simulink model "simulink_app"  (R2015a)
settings: Solver=ode2  SolverMode=SingleTasking  StartTime=0.0  StopTime=inf  FixedStep=T_ctrl  RelTol=1e-3
undefined symbols (not defined in the file): A_l_max_x, A_l_max_y, A_z_max, B_hover_4dof, CG_0, epsilon, eta_23, g, h, h_M, Hover_eta_23, Hover_throtle_1, Hover_throtle_23, I_BAC_0, Ix, Iy, Iz, l, l_arm, m, m_0, m_M, Rotation_sign, T_ctrl, throtle_1, throtle_23, v_i0
libraries: XXCopter_Control x52, simulink x11, XXCopter x1
(part 2 of 4)

== system simulink_app/Control and guidance/Otter Overactuated P Controller ==
  Position ref (m) : Inport
  Vel_yaw_ref(m) : Inport  Port=2
  All meas : Inport  Port=3
  activation_bus : Inport  Port=4
  init_cond : Inport  Port=5
  AWU : Product  Multiplication=Matrix(*)
  Add : Sum
  Add1 : Sum  Inputs=+-
  Add2 : Sum  Inputs=+-
  Bus Selector1 : BusSelector  OutputSignals=Params.T_Fe_Fyaw,Params.V_yaw,Params.DCM
  Bus Selector2 : BusSelector  OutputSignals=pos_xy_act,vel_yaw_xy_act,alt_act,vel_yaw_z_act
  Demux1 : Demux  Outputs=3
  Demux2 : Demux  Outputs=3
  Demux3 : Demux  Outputs=[2,1]
  Logical Operator : Logic  IconShape=distinctive  AllPortsSameDT=off  OutDataTypeStr=boolean
  Logical Operator1 : Logic  Operator=NOT  IconShape=distinctive  AllPortsSameDT=off  OutDataTypeStr=boolean
  Logical Operator2 : Logic  Operator=NOT  IconShape=distinctive  AllPortsSameDT=off  OutDataTypeStr=boolean
  Logical Operator3 : Logic  IconShape=distinctive  AllPortsSameDT=off  OutDataTypeStr=boolean
  Matrix Multiply1 : Product  Multiplication=Matrix(*)
  Matrix Multiply2 : Product  Multiplication=Matrix(*)
  Matrix Multiply3 : Product  Multiplication=Matrix(*)
  Memory : Memory  X0=[0;0;0]  InheritSampleTime=on
  Mux : Mux  Inputs=[2,1]
  Permute Dimensions : PermuteDimensions
  Permute Dimensions1 : PermuteDimensions
  Permute Dimensions2 : PermuteDimensions
  Position Controller : Subsystem
  Saturation : Saturate  UpperLimit=[A_l_max_x,A_l_max_y,g]  LowerLimit=-[A_l_max_x,A_l_max_y,A_z_max-g]
  Saturation1 : Saturate  UpperLimit=[10,10,v_i0]'  LowerLimit=-[10,10,2*v_i0]'
  Selector : Selector  InputPortWidth=3  Indices=[1,2]
  Selector1 : Selector  InputPortWidth=3  Indices=3
  Switch : Switch  Criteria=u2 ~= 0
  Switch1 : Switch  Criteria=u2 ~= 0
  T : Gain  Gain=T_ctrl
  Velocity Controller : Subsystem
  activation_bus1 : InportShadow  Port=4
  init_cond1 : InportShadow  Port=5
  Accels des : Outport
  wires:
  Demux2/3 -> Velocity Controller/3(Vyaw_z_ref)
  Demux2/1 -> Velocity Controller/1(Vyaw_x_ref)
  Demux2/2 -> Velocity Controller/2(Vyaw_y_ref)
  All meas/1 -> Position Controller/6(All_meas), Bus Selector1/1
  Position ref (m)/1 -> Demux1/1
  Demux1/3 -> Position Controller/4(X_e_z_ref)
  Demux1/2 -> Position Controller/3(X_e_y_ref)
  Demux1/1 -> Position Controller/2(X_e_x_ref)
  Bus Selector1/3 -> Permute Dimensions/1  "<DCM>"
  Matrix Multiply1/1 -> Accels des/1
  Permute Dimensions/1 -> Matrix Multiply1/1
  Position Controller/1(Ve des (m/s)) -> Matrix Multiply2/2
  Saturation1/1 -> Add1/1, Demux2/1
  Saturation/1 -> Add2/1, Matrix Multiply3/2
  Bus Selector1/1 -> Permute Dimensions2/1, Matrix Multiply2/1, Permute Dimensions1/1  "<T_Fe_Fyaw>"
  Mux/1 -> Add1/2, Saturation1/1
  Matrix Multiply3/1 -> Matrix Multiply1/2  "in F_e"
  Permute Dimensions1/1 -> Matrix Multiply3/1
  Velocity Controller/1(Acc_yaw des (m/s)) -> Add2/2, Saturation/1
  Permute Dimensions2/1 -> AWU/1
  Add/1 -> AWU/2
  Add2/1 -> T/1
  Add1/1 -> Add/2
  AWU/1 -> Memory/1
  T/1 -> Add/1
  activation_bus/1 -> Bus Selector2/1, Position Controller/5(activation_bus)
  activation_bus1/1 -> Velocity Controller/5(activation_bus)
  init_cond/1 -> Position Controller/7(init_cond)
  Bus Selector1/2 -> Velocity Controller/4(V_yaw_meas)  "<V_yaw>"
  Matrix Multiply2/1 -> Demux3/1
  Switch/1 -> Mux/1
  Demux3/1 -> Switch/3
  Vel_yaw_ref(m)/1 -> Selector/1, Selector1/1
  Selector/1 -> Switch/1
  Switch1/1 -> Mux/2
  Demux3/2 -> Switch1/3
  Selector1/1 -> Switch1/1
  init_cond1/1 -> Velocity Controller/6(Init_cond)
  Bus Selector2/1 -> Logical Operator1/1  "<pos_xy_act>"
  Bus Selector2/3 -> Logical Operator2/1  "<alt_act>"
  Logical Operator1/1 -> Logical Operator/1
  Bus Selector2/2 -> Logical Operator/2  "<vel_yaw_xy_act>"
  Logical Operator2/1 -> Logical Operator3/1
  Bus Selector2/4 -> Logical Operator3/2  "<vel_yaw_z_act>"
  Logical Operator/1 -> Switch/2
  Logical Operator3/1 -> Switch1/2
  Memory/1 -> Position Controller/1(AWU)

== system simulink_app/Control and guidance/keep -90//90 ==
  in (rad) : Inport
  Constant : Constant  Value=180
  Constant2 : Constant  Value=360
  Gain : Gain  Gain=360
  Math Function2 : Math  Operator=rem  SaturateOnIntegerOverflow=on
  Product : Product  Inputs=*/  RndMeth=Zero
  Rounding Function : Rounding  Operator=fix
  Sum2 : Sum  Inputs=|-+
  deg2rad1 : Gain  Gain=pi/180  SaturateOnIntegerOverflow=on  OutDataTypeStr=Inherit: Same as input  ParamDataTypeStr=Inherit: Same as input
  rad2deg : Gain  Gain=180/pi  SaturateOnIntegerOverflow=on  OutDataTypeStr=Inherit: Same as input  ParamDataTypeStr=Inherit: Same as input
  out (rad) : Outport
  wires:
  deg2rad1/1 -> out (rad)/1
  Sum2/1 -> deg2rad1/1
  Math Function2/1 -> Sum2/2, Product/1
  Constant2/1 -> Math Function2/2
  rad2deg/1 -> Math Function2/1
  Gain/1 -> Sum2/1
  Rounding Function/1 -> Gain/1
  Product/1 -> Rounding Function/1
  Constant/1 -> Product/2
  in (rad)/1 -> rad2deg/1

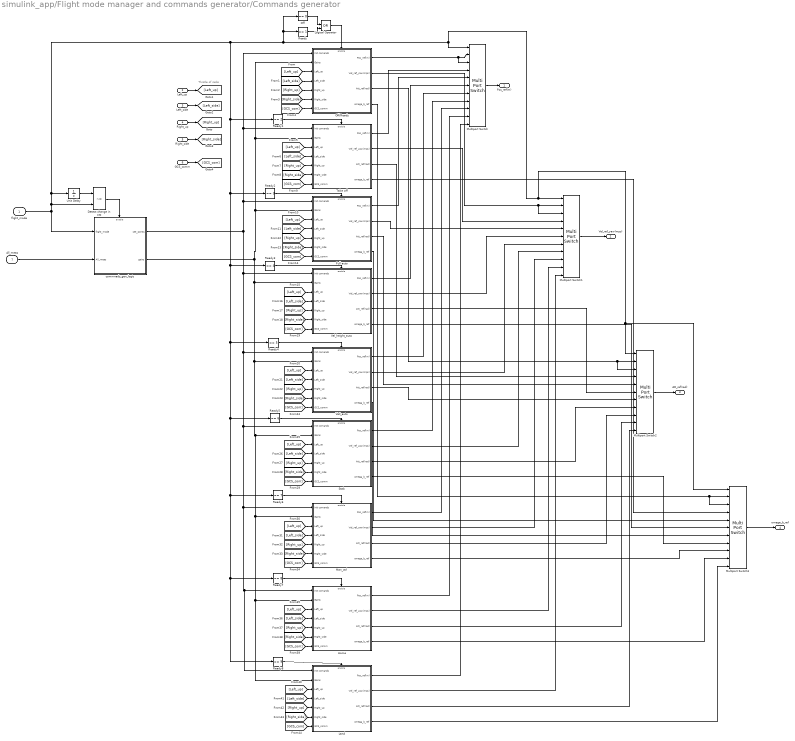
== system simulink_app/Flight mode manager and commands generator/Commands generator ==
  note: Throtle of radio
  flight_mode : Inport
  Left_up : Inport  Port=2
  Left_side : Inport  Port=3
  Right_up : Inport  Port=4
  Right_side : Inport  Port=5
  GCS_comm : Inport  Port=6
  All_meas : Inport  Port=7
  Detect change in FM : RelationalOperator  Operator=~=  OutDataTypeStr=boolean
  Full auto : Subsystem  TreatAsAtomicUnit=on
  Home : Subsystem  TreatAsAtomicUnit=on
  "Land " : Subsystem  TreatAsAtomicUnit=on
  Logical Operator : Logic  Operator=OR  IconShape=distinctive  AllPortsSameDT=off  OutDataTypeStr=boolean
  Man_ctrl : Subsystem  TreatAsAtomicUnit=on
  Multiport Switch{,1..3} (4 alike) : MultiPortSwitch  DataPortOrder=Zero-based contiguous  Inputs=10
  Off : simulink/Logic and Bit Operations/Compare To Constant  relop===  const=0  OutDataTypeStr=boolean
  Off/Ready : Subsystem  TreatAsAtomicUnit=on
  Ready : simulink/Logic and Bit Operations/Compare To Constant  relop===  const=1  OutDataTypeStr=boolean
  Ready1 : simulink/Logic and Bit Operations/Compare To Constant  relop===  const=2  OutDataTypeStr=boolean
  Ready2 : simulink/Logic and Bit Operations/Compare To Constant  relop===  const=3  OutDataTypeStr=boolean
  Ready3 : simulink/Logic and Bit Operations/Compare To Constant  relop===  const=4  OutDataTypeStr=boolean
  Ready4 : simulink/Logic and Bit Operations/Compare To Constant  relop===  const=5  OutDataTypeStr=boolean
  Ready5 : simulink/Logic and Bit Operations/Compare To Constant  relop===  const=6  OutDataTypeStr=boolean
  Ready6 : simulink/Logic and Bit Operations/Compare To Constant  relop===  const=7  OutDataTypeStr=boolean
  Ready7 : simulink/Logic and Bit Operations/Compare To Constant  relop===  const=8  OutDataTypeStr=boolean
  Ready8 : simulink/Logic and Bit Operations/Compare To Constant  relop===  const=9  OutDataTypeStr=boolean
  Stab : Subsystem  TreatAsAtomicUnit=on
  Take off : Subsystem  TreatAsAtomicUnit=on
  Unit Delay : UnitDelay  SampleTime=-1
  Vel_height_auto : Subsystem  TreatAsAtomicUnit=on
  Vell_auto : Subsystem  TreatAsAtomicUnit=on
  commnads_gen_logic : Subsystem
  Pos_ref(m) : Outport
  Vel_ref_yaw(mps) : Outport  Port=2
  Att_ref(rad) : Outport  Port=3
  omega_b_ref : Outport  Port=4
  wires:
  flight_mode/1 -> Detect change in FM/2, Unit Delay/1, Ready8/1, Ready7/1, Ready6/1, Ready5/1, Ready4/1, Ready3/1, Ready2/1, Ready1/1, Ready/1, Off/1, Multiport Switch2/1, Multiport Switch3/1, Multiport Switch1/1, Multiport Switch/1, commnads_gen_logic/1(flight_mode)
  Multiport Switch/1 -> Pos_ref(m)/1
  Multiport Switch1/1 -> Vel_ref_yaw(mps)/1
  Multiport Switch2/1 -> Att_ref(rad)/1
  Multiport Switch3/1 -> omega_b_ref/1
  Right_up/1 -> [Right_up]
  Left_up/1 -> [Left_up]
  Right_side/1 -> [Right_side]
  Left_side/1 -> [Left_side]
  GCS_comm/1 -> [GCS_com]
  [Left_up] -> Off/Ready/3(Left_up)
  [Left_side] -> Off/Ready/4(Left_side)
  [Right_up] -> Off/Ready/5(Right_up)
  [Right_side] -> Off/Ready/6(Right_side)
  [GCS_com] -> Off/Ready/7(GCS_comm)
  [Left_up] -> Take off/3(Left_up)
  [Left_side] -> Take off/4(Left_side)
  [Right_up] -> Take off/5(Right_up)
  [Right_side] -> Take off/6(Right_side)
  [GCS_com] -> Take off/7(GCS_comm)
  [Left_up] -> Full auto/3(Left_up)
  [Left_side] -> Full auto/4(Left_side)
  [Right_up] -> Full auto/5(Right_up)
  [Right_side] -> Full auto/6(Right_side)
  [GCS_com] -> Full auto/7(GCS_comm)
  [Left_up] -> Vel_height_auto/3(Left_up)
  [Left_side] -> Vel_height_auto/4(Left_side)
  [Right_up] -> Vel_height_auto/5(Right_up)
  [Right_side] -> Vel_height_auto/6(Right_side)
  [GCS_com] -> Vel_height_auto/7(GCS_comm)
  [Left_up] -> Vell_auto/3(Left_up)
  [Left_side] -> Vell_auto/4(Left_side)
  [Right_up] -> Vell_auto/5(Right_up)
  [Right_side] -> Vell_auto/6(Right_side)
  [GCS_com] -> Vell_auto/7(GCS_comm)
  [Left_up] -> Stab/3(Left_up)
  [Left_side] -> Stab/4(Left_side)
  [Right_up] -> Stab/5(Right_up)
  [Right_side] -> Stab/6(Right_side)
  [GCS_com] -> Stab/7(GCS_comm)
  [Left_up] -> Man_ctrl/3(Left_up)
  [Left_side] -> Man_ctrl/4(Left_side)
  [Right_up] -> Man_ctrl/5(Right_up)
  [Right_side] -> Man_ctrl/6(Right_side)
  [GCS_com] -> Man_ctrl/7(GCS_comm)
  [Left_up] -> Home/3(Left_up)
  [Left_side] -> Home/4(Left_side)
  [Right_up] -> Home/5(Right_up)
  [Right_side] -> Home/6(Right_side)
  [GCS_com] -> Home/7(GCS_comm)
  [Left_up] -> "Land "/3(Left_up)
  [Left_side] -> "Land "/4(Left_side)
  [Right_up] -> "Land "/5(Right_up)
  [Right_side] -> "Land "/6(Right_side)
  [GCS_com] -> "Land "/7(GCS_comm)
  Off/1 -> Logical Operator/1
  Ready/1 -> Logical Operator/2
  Logical Operator/1 -> Off/Ready/Enable
  Ready1/1 -> Take off/Enable
  Ready2/1 -> Full auto/Enable
  Ready3/1 -> Vel_height_auto/Enable
  Ready4/1 -> Vell_auto/Enable
  Ready5/1 -> Stab/Enable
  Ready6/1 -> Man_ctrl/Enable
  Ready7/1 -> Home/Enable
  Ready8/1 -> "Land "/Enable
  Off/Ready/1(Pos_ref(m)) -> Multiport Switch/3, Multiport Switch/2
  Take off/1(Pos_ref(m)) -> Multiport Switch/4
  Full auto/1(Pos_ref(m)) -> Multiport Switch/5
  Vel_height_auto/1(Pos_ref(m)) -> Multiport Switch/6
  Vell_auto/1(Pos_ref(m)) -> Multiport Switch/7
  Stab/1(Pos_ref(m)) -> Multiport Switch/8
  Man_ctrl/1(Pos_ref(m)) -> Multiport Switch/9
  Home/1(Pos_ref(m)) -> Multiport Switch/10
  "Land "/1(Pos_ref(m)) -> Multiport Switch/11
  Off/Ready/2(Vel_ref_yaw(mps)) -> Multiport Switch1/3, Multiport Switch1/2
  Take off/2(Vel_ref_yaw(mps)) -> Multiport Switch1/4
  Full auto/2(Vel_ref_yaw(mps)) -> Multiport Switch1/5
  Vel_height_auto/2(Vel_ref_yaw(mps)) -> Multiport Switch1/6
  Vell_auto/2(Vel_ref_yaw(mps)) -> Multiport Switch1/7
  Stab/2(Vel_ref_yaw(mps)) -> Multiport Switch1/8
  Man_ctrl/2(Vel_ref_yaw(mps)) -> Multiport Switch1/9
  Home/2(Vel_ref_yaw(mps)) -> Multiport Switch1/10
  "Land "/2(Vel_ref_yaw(mps)) -> Multiport Switch1/11
  Off/Ready/3(Att_ref(rad)) -> Multiport Switch2/3, Multiport Switch2/2
  Take off/3(Att_ref(rad)) -> Multiport Switch2/4
  Full auto/3(Att_ref(rad)) -> Multiport Switch2/5
  Vel_height_auto/3(Att_ref(rad)) -> Multiport Switch2/6
  Vell_auto/3(Att_ref(rad)) -> Multiport Switch2/7
  Stab/3(Att_ref(rad)) -> Multiport Switch2/8
  Man_ctrl/3(Att_ref(rad)) -> Multiport Switch2/9
  Home/3(Att_ref(rad)) -> Multiport Switch2/10
  "Land "/3(Att_ref(rad)) -> Multiport Switch2/11
  Off/Ready/4(omega_b_ref) -> Multiport Switch3/3, Multiport Switch3/2
  Take off/4(omega_b_ref) -> Multiport Switch3/4
  Full auto/4(omega_b_ref) -> Multiport Switch3/5
  Vel_height_auto/4(omega_b_ref) -> Multiport Switch3/6
  Vell_auto/4(omega_b_ref) -> Multiport Switch3/7
  Stab/4(omega_b_ref) -> Multiport Switch3/8
  Man_ctrl/4(omega_b_ref) -> Multiport Switch3/9
  Home/4(omega_b_ref) -> Multiport Switch3/10
  "Land "/4(omega_b_ref) -> Multiport Switch3/11
  commnads_gen_logic/2(gains) -> Full auto/2(Gains), Take off/2(Gains), Off/Ready/2(Gains), Stab/2(Gains), "Land "/2(Gains), Home/2(Gains), Man_ctrl/2(Gains), Vell_auto/2(Gains), Vel_height_auto/2(Gains)
  commnads_gen_logic/1(set_points) -> Take off/1(Init comands), Off/Ready/1(Init comands), Full auto/1(Init comands), Stab/1(Init comands), "Land "/1(Init comands), Home/1(Init comands), Man_ctrl/1(Init comands), Vell_auto/1(Init comands), Vel_height_auto/1(Init comands)
  All_meas/1 -> commnads_gen_logic/2(All_meas)
  Unit Delay/1 -> Detect change in FM/1
  Detect change in FM/1 -> commnads_gen_logic/Enable

== system simulink_app/Flight mode manager and commands generator/Flight manager ==
  note: This guy should be able to overwrite any flghlit_mode at any moment
  flight_mode_request : Inport
  All_meas : Inport  Port=2
  Safety_stab_switch : Inport  Port=3
  Bus Selector : BusSelector  OutputSignals=Params.gps_pdop,Params.gps_sat,Meas.Pos_meas_m,Params.V_yaw,Meas.Eulr_meas_rad,Meas.Volt
  Bus Selector1 : BusSelector  OutputSignals=Params.gps_pdop,Params.gps_vdop,Params.gps_sat,Meas.Pos_meas_m,Meas.Volt,Params.a_meas
  Memory : Memory
  Parameters_based_decision_making : MATLAB Function  TreatAsAtomicUnit=on
  Selector : Selector  InputPortWidth=3  Indices=3
  Unary Minus : UnaryMinus
  flight_mode_manager : MATLAB Function  TreatAsAtomicUnit=on
  flight_mode : Outport
  not_allowed_transition : Outport  Port=2
  wires:
  flight_mode_request/1 -> flight_mode_manager/1(flight_mode_reqest)
  All_meas/1 -> Bus Selector1/1, Bus Selector/1
  flight_mode_manager/1(flight_mode_out) -> Parameters_based_decision_making/1(flight_mode)
  Parameters_based_decision_making/1(flight_mode_out) -> flight_mode/1, Memory/1
  Memory/1 -> flight_mode_manager/9(flight_mode)
  Safety_stab_switch/1 -> flight_mode_manager/2(Safety_stab_switch)
  Bus Selector/1 -> flight_mode_manager/3(p_dop)  "<gps_pdop>"
  Bus Selector/5 -> flight_mode_manager/7(Euler)  "<Eulr_meas_rad>"
  Bus Selector/4 -> flight_mode_manager/6(Vyaw)  "<V_yaw>"
  Bus Selector/3 -> flight_mode_manager/5(Xe)  "<Pos_meas_m>"
  Bus Selector/2 -> flight_mode_manager/4(num_sats)  "<gps_sat>"
  Bus Selector1/1 -> Parameters_based_decision_making/2(pdop)  "<gps_pdop>"
  Bus Selector1/2 -> Parameters_based_decision_making/3(vdop)  "<gps_vdop>"
  Bus Selector1/3 -> Parameters_based_decision_making/4(num_sats)  "<gps_sat>"
  Bus Selector1/5 -> Parameters_based_decision_making/6(Volt)  "<Volt>"
  Bus Selector1/6 -> Parameters_based_decision_making/7(Accs)  "<a_meas>"
  Selector/1 -> Unary Minus/1
  Bus Selector1/4 -> Selector/1  "<Pos_meas_m>"
  Unary Minus/1 -> Parameters_based_decision_making/5(Alt)
  Bus Selector/6 -> flight_mode_manager/8(Volt)  "<Volt>"
  flight_mode_manager/2(NOT_allowed_sign) -> not_allowed_transition/1

== system simulink_app/Px4_to_simulink input interface/DCM1 ==
  Euler : Inport  PortDimensions=3
  Fcn11 : Fcn  Expr=u(5)*u(4)
  Fcn12 : Fcn  Expr=u(5)*u(1)
  Fcn13 : Fcn  Expr=-u(2)
  Fcn21 : Fcn  Expr=u(3)*u(2)*u(4) - u(6)*u(1)
  Fcn22 : Fcn  Expr=u(3)*u(2)*u(1) + u(6)*u(4)
  Fcn23 : Fcn  Expr=u(3)*u(5)
  Fcn31 : Fcn  Expr=u(6)*u(2)*u(4) + u(3)*u(1)
  Fcn32 : Fcn  Expr=u(6)*u(2)*u(1) - u(3)*u(4)
  Fcn33 : Fcn  Expr=u(6)*u(5)
  Mux : Mux  Inputs=2
  Mux1 : Mux  Inputs=9
  Reshape : Reshape  OutputDimensionality=Customize  OutputDimensions=[3,3]
  sincos : Trigonometry  Operator=sincos
  DCM : Outport  PortDimensions=[3,3]
  wires:
  Fcn33/1 -> Mux1/9
  Fcn32/1 -> Mux1/8
  Fcn23/1 -> Mux1/6
  Fcn22/1 -> Mux1/5
  Fcn31/1 -> Mux1/7
  Fcn21/1 -> Mux1/4
  Fcn13/1 -> Mux1/3
  Fcn12/1 -> Mux1/2
  Fcn11/1 -> Mux1/1
  Mux/1 -> Fcn22/1, Fcn23/1, Fcn31/1, Fcn33/1, Fcn32/1, Fcn21/1, Fcn13/1, Fcn12/1, Fcn11/1
  sincos/2 -> Mux/2
  sincos/1 -> Mux/1
  Reshape/1 -> DCM/1
  Euler/1 -> sincos/1
  Mux1/1 -> Reshape/1

== system simulink_app/Control and guidance/Control allocator/Hover deflections1 ==
  Contro Inputs1 : Constant  Value=Hover_throtle_1
  Contro Inputs2 : Constant  Value=Hover_throtle_23
  Contro Inputs3 : Constant  Value=Hover_eta_23
  Gain : Gain  Gain=-1
  Ground : Ground
  Mux : Mux  Inputs=9
  Trim deflectins : Outport
  wires:
  Contro Inputs1/1 -> Mux/1
  Contro Inputs2/1 -> Mux/7, Mux/4
  Ground/1 -> Mux/2, Mux/6, Mux/9, Mux/3
  Contro Inputs3/1 -> Gain/1, Mux/5
  Gain/1 -> Mux/8
  Mux/1 -> Trim deflectins/1

== system simulink_app/Control and guidance/Control allocator/Hover deflections2 ==
  Contro Inputs1 : Constant  Value=Hover_throtle_1
  Contro Inputs2 : Constant  Value=Hover_throtle_23
  Contro Inputs3 : Constant  Value=Hover_eta_23
  Gain : Gain  Gain=-1
  Ground : Ground
  Mux : Mux  Inputs=9
  Trim deflectins : Outport
  wires:
  Contro Inputs1/1 -> Mux/1
  Contro Inputs2/1 -> Mux/7, Mux/4
  Ground/1 -> Mux/2, Mux/6, Mux/9, Mux/3
  Contro Inputs3/1 -> Gain/1, Mux/5
  Gain/1 -> Mux/8
  Mux/1 -> Trim deflectins/1

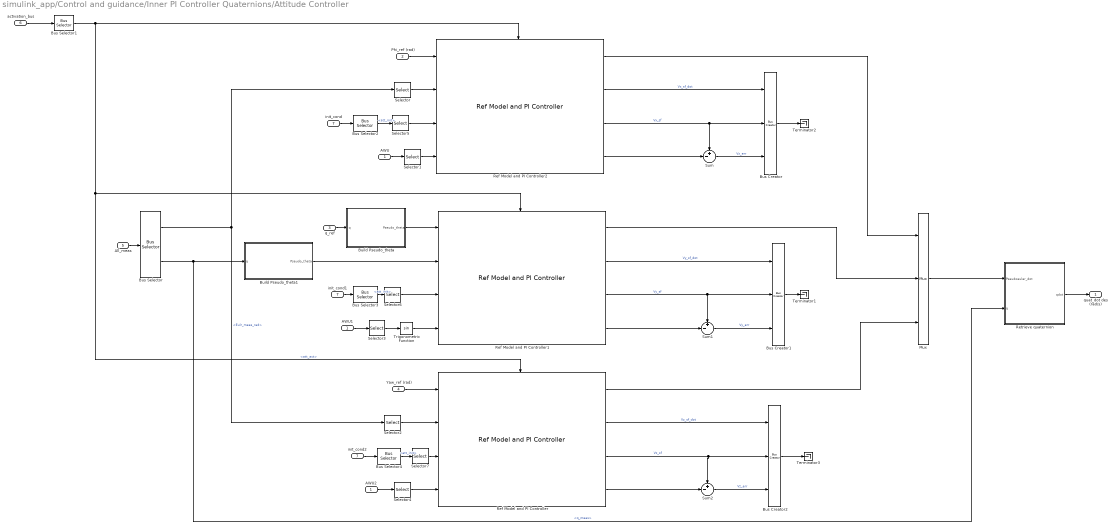
== system simulink_app/Control and guidance/Inner PI Controller Quaternions/Attitude Controller ==
  AWU : Inport
  Phi_ref (rad) : Inport  Port=2
  q_ref : Inport  Port=3
  Yaw_ref (rad) : Inport  Port=4
  All_meas : Inport  Port=5
  activation_bus : Inport  Port=6
  init_cond : Inport  Port=7
  AWU1 : InportShadow
  AWU2 : InportShadow
  Build Pseudo_theta : MATLAB Function  TreatAsAtomicUnit=on
  Build Pseudo_theta1 : MATLAB Function  TreatAsAtomicUnit=on
  Bus Creator : BusCreator  Inputs=3
  Bus Creator1 : BusCreator  Inputs=3
  Bus Creator2 : BusCreator  Inputs=3
  Bus Selector : BusSelector  OutputSignals=Meas.Eulr_meas_rad,Meas.q_meas
  Bus Selector1 : BusSelector  OutputSignals=att_act
  Bus Selector2 : BusSelector  OutputSignals=att_init
  Bus Selector3 : BusSelector  OutputSignals=att_init
  Bus Selector4 : BusSelector  OutputSignals=att_init
  Mux : Mux  Inputs=3
  Ref Model and PI Controller : XXCopter_Control/Ref Model and PI Controller  delta=0  tau=2  RisingSlewLimit=deg2rad(8)  FallingSlewLimit=-deg2rad(8)  K_f=0  K_a=1  Con_way=pro  omega_n=4  xi=0.5  Z1=-30  K_b=2  f_i=0.15  f_c=1
  Ref Model and PI Controller1 : XXCopter_Control/Ref Model and PI Controller  delta=0  tau=1.5  RisingSlewLimit=deg2rad(8)  FallingSlewLimit=-deg2rad(8)  K_f=0  K_a=1  Con_way=pro  omega_n=4  xi=0.5  Z1=-30  K_b=1.2  f_i=0.1  f_c=1
  Ref Model and PI Controller2 : XXCopter_Control/Ref Model and PI Controller  delta=0  tau=1.5  RisingSlewLimit=deg2rad(8)  FallingSlewLimit=-deg2rad(8)  K_f=0  K_a=1  Con_way=pro  omega_n=4  xi=0.5  Z1=-30  K_b=1.5  f_i=0.1  f_c=1
  Retrieve quaternion : MATLAB Function  TreatAsAtomicUnit=on
  Selector : Selector  InputPortWidth=3
  Selector1 : Selector  InputPortWidth=3
  Selector2 : Selector  InputPortWidth=3  Indices=3
  Selector3 : Selector  InputPortWidth=3  Indices=2
  Selector4 : Selector  InputPortWidth=3  Indices=3
  Selector5 : Selector  InputPortWidth=3
  Selector6 : Selector  InputPortWidth=3  Indices=2
  Selector7 : Selector  InputPortWidth=3  Indices=3
  Sum : Sum  Inputs=+-|
  Sum1 : Sum  Inputs=+-|
  Sum2 : Sum  Inputs=+-|
  Terminator1 : Terminator
  Terminator2 : Terminator
  Terminator3 : Terminator
  Trigonometric Function : Trigonometry
  init_cond1 : InportShadow  Port=7
  init_cond2 : InportShadow  Port=7
  quat_dot des (rad/s) : Outport
  wires:
  Ref Model and PI Controller/4 -> Sum2/2
  Sum2/1 -> Bus Creator2/3  "Vz_err"
  Ref Model and PI Controller/3 -> Bus Creator2/2, Sum2/1  "Vz_sf"
  Ref Model and PI Controller/2 -> Bus Creator2/1  "Vz_sf_dot"
  Ref Model and PI Controller1/4 -> Sum1/2
  Sum1/1 -> Bus Creator1/3  "Vy_err"
  Ref Model and PI Controller1/3 -> Bus Creator1/2, Sum1/1  "Vy_sf"
  Ref Model and PI Controller1/2 -> Bus Creator1/1  "Vy_sf_dot"
  Ref Model and PI Controller2/4 -> Sum/2
  Bus Creator2/1 -> Terminator3/1
  Bus Creator1/1 -> Terminator1/1
  Bus Creator/1 -> Terminator2/1
  Sum/1 -> Bus Creator/3  "Vx_err"
  Ref Model and PI Controller2/3 -> Bus Creator/2, Sum/1  "Vx_sf"
  Ref Model and PI Controller2/2 -> Bus Creator/1  "Vx_sf_dot"
  Yaw_ref (rad)/1 -> Ref Model and PI Controller/1
  Selector/1 -> Ref Model and PI Controller2/2
  Bus Selector/2 -> Retrieve quaternion/2(q), Build Pseudo_theta1/1(q)  "<q_meas>"
  All_meas/1 -> Bus Selector/1
  q_ref/1 -> Build Pseudo_theta/1(q)
  Phi_ref (rad)/1 -> Ref Model and PI Controller2/1
  Retrieve quaternion/1(qdot) -> quat_dot des (rad/s)/1
  Ref Model and PI Controller2/1 -> Mux/1
  Ref Model and PI Controller/1 -> Mux/3
  Ref Model and PI Controller1/1 -> Mux/2
  Mux/1 -> Retrieve quaternion/1(Pseudoeuler_dot)
  Selector2/1 -> Ref Model and PI Controller/2
  Bus Selector/1 -> Selector2/1, Selector/1  "<Eulr_meas_rad>"
  Build Pseudo_theta1/1(Pseudo_theta) -> Ref Model and PI Controller1/2
  Build Pseudo_theta/1(Pseudo_theta) -> Ref Model and PI Controller1/1
  AWU/1 -> Selector1/1
  AWU1/1 -> Selector3/1
  AWU2/1 -> Selector4/1
  Selector3/1 -> Trigonometric Function/1
  Selector1/1 -> Ref Model and PI Controller2/4
  Trigonometric Function/1 -> Ref Model and PI Controller1/4
  Selector4/1 -> Ref Model and PI Controller/4
  activation_bus/1 -> Bus Selector1/1
  Bus Selector1/1 -> Ref Model and PI Controller/Enable, Ref Model and PI Controller1/Enable, Ref Model and PI Controller2/Enable  "<att_act>"
  init_cond/1 -> Bus Selector2/1
  Bus Selector2/1 -> Selector5/1  "<att_init>"
  Selector5/1 -> Ref Model and PI Controller2/3
  Selector6/1 -> Ref Model and PI Controller1/3
  init_cond1/1 -> Bus Selector3/1
  Bus Selector3/1 -> Selector6/1  "<att_init>"
  init_cond2/1 -> Bus Selector4/1
  Selector7/1 -> Ref Model and PI Controller/3
  Bus Selector4/1 -> Selector7/1  "<att_init>"

== system simulink_app/Control and guidance/Inner PI Controller Quaternions/Body Rates Controller ==
  p_ref : Inport
  q_ref : Inport  Port=2
  r_ref : Inport  Port=3
  All_meas : Inport  Port=4
  init_cond : Inport  Port=5
  activation_bus : Inport  Port=6
  Bus Creator : BusCreator
  Bus Creator1 : BusCreator
  Bus Creator2 : BusCreator
  Bus Selector : BusSelector  OutputSignals=Meas.omega_b_meas_radps
  Bus Selector1 : BusSelector  OutputSignals=omega_b_act
  Bus Selector2 : BusSelector  OutputSignals=b_rates_init
  Bus Selector3 : BusSelector  OutputSignals=b_rates_init
  Bus Selector4 : BusSelector  OutputSignals=b_rates_init
  Mux : Mux  Inputs=3
  Ref Model and P Controller p : XXCopter_Control/Ref Model and P Controller  tau=0.7  RisingSlewLimit=4  FallingSlewLimit=-4  K_f=0.7  K_b=6
  Ref Model and P Controller q : XXCopter_Control/Ref Model and P Controller  tau=0.7  RisingSlewLimit=4  FallingSlewLimit=-4  K_f=0.7  K_b=6
  Ref Model and P Controller r : XXCopter_Control/Ref Model and P Controller  tau=1.5  RisingSlewLimit=4  FallingSlewLimit=-4  K_f=0.7  K_b=1.5
  Selector : Selector  InputPortWidth=3
  Selector1 : Selector  InputPortWidth=3  Indices=2
  Selector2 : Selector  InputPortWidth=3  Indices=3
  Selector3 : Selector  InputPortWidth=3
  Selector4 : Selector  InputPortWidth=3  Indices=2
  Selector5 : Selector  InputPortWidth=3  Indices=3
  Sum : Sum  Inputs=+-|
  Sum1 : Sum  Inputs=+-|
  Sum2 : Sum  Inputs=+-|
  Terminator1 : Terminator
  Terminator2 : Terminator
  Terminator3 : Terminator
  init_cond1 : InportShadow  Port=5
  init_cond2 : InportShadow  Port=5
  Angular acc des (rad/s^2) : Outport
  wires:
  Ref Model and P Controller r/5 -> Bus Creator2/4  "K_b_r"
  Ref Model and P Controller r/4 -> Sum2/2
  Sum2/1 -> Bus Creator2/3  "r_err"
  Ref Model and P Controller r/3 -> Bus Creator2/2, Sum2/1  "r_sf"
  Ref Model and P Controller r/2 -> Bus Creator2/1  "r_sf_dot"
  Ref Model and P Controller q/5 -> Bus Creator1/4  "K_b_q"
  Ref Model and P Controller q/4 -> Sum1/2
  Sum1/1 -> Bus Creator1/3  "q_err"
  Ref Model and P Controller q/3 -> Bus Creator1/2, Sum1/1  "q_sf"
  Ref Model and P Controller q/2 -> Bus Creator1/1  "q_sf_dot"
  Ref Model and P Controller p/5 -> Bus Creator/4  "K_b_p"
  Ref Model and P Controller p/4 -> Sum/2
  Selector2/1 -> Ref Model and P Controller r/2
  Bus Creator2/1 -> Terminator3/1
  Bus Creator1/1 -> Terminator1/1
  Bus Creator/1 -> Terminator2/1
  Sum/1 -> Bus Creator/3  "p_err"
  Ref Model and P Controller p/3 -> Bus Creator/2, Sum/1  "p_sf"
  Ref Model and P Controller p/2 -> Bus Creator/1  "p_sf_dot"
  r_ref/1 -> Ref Model and P Controller r/1
  Selector1/1 -> Ref Model and P Controller q/2
  q_ref/1 -> Ref Model and P Controller q/1
  Mux/1 -> Angular acc des (rad/s^2)/1
  p_ref/1 -> Ref Model and P Controller p/1
  Bus Selector/1 -> Selector2/1, Selector/1, Selector1/1  "<omega_b_meas_radps>"
  All_meas/1 -> Bus Selector/1
  Ref Model and P Controller r/1 -> Mux/3
  Ref Model and P Controller q/1 -> Mux/2
  Ref Model and P Controller p/1 -> Mux/1
  Selector/1 -> Ref Model and P Controller p/2
  activation_bus/1 -> Bus Selector1/1
  Bus Selector1/1 -> Ref Model and P Controller p/Enable, Ref Model and P Controller r/Enable, Ref Model and P Controller q/Enable  "<omega_b_act>"
  init_cond/1 -> Bus Selector2/1
  Bus Selector2/1 -> Selector3/1  "<b_rates_init>"
  Selector3/1 -> Ref Model and P Controller p/3
  init_cond1/1 -> Bus Selector3/1
  Bus Selector3/1 -> Selector4/1  "<b_rates_init>"
  Selector4/1 -> Ref Model and P Controller q/3
  init_cond2/1 -> Bus Selector4/1
  Bus Selector4/1 -> Selector5/1  "<b_rates_init>"
  Selector5/1 -> Ref Model and P Controller r/3

== system simulink_app/Control and guidance/Inner PI Controller Quaternions/Limits in Ang accel ==
  note: Here it is assumed that at all time every prop is generating m*g/3 newtons of force . It is conservative?
  Ang Ace des : Inport
  Euler meas : Inport  Port=2
  Limis eval : MATLAB Function  TreatAsAtomicUnit=on
  Saturation Dynamic : simulink/Discontinuities/Saturation Dynamic  OutMin=[]  OutMax=[]  OutDataTypeStr=Inherit: Same as second input  OutDataType=fixdt(1, 16)  OutScaling=2^-10  DoSatur=off
  ang Ace des : Outport
  wires:
  Limis eval/1(Limit_up) -> Saturation Dynamic/1
  Limis eval/2(Limit_down) -> Saturation Dynamic/3
  Euler meas/1 -> Limis eval/2(euler_ang)
  Ang Ace des/1 -> Saturation Dynamic/2, Limis eval/1(Ang_Accel)
  Saturation Dynamic/1 -> ang Ace des/1

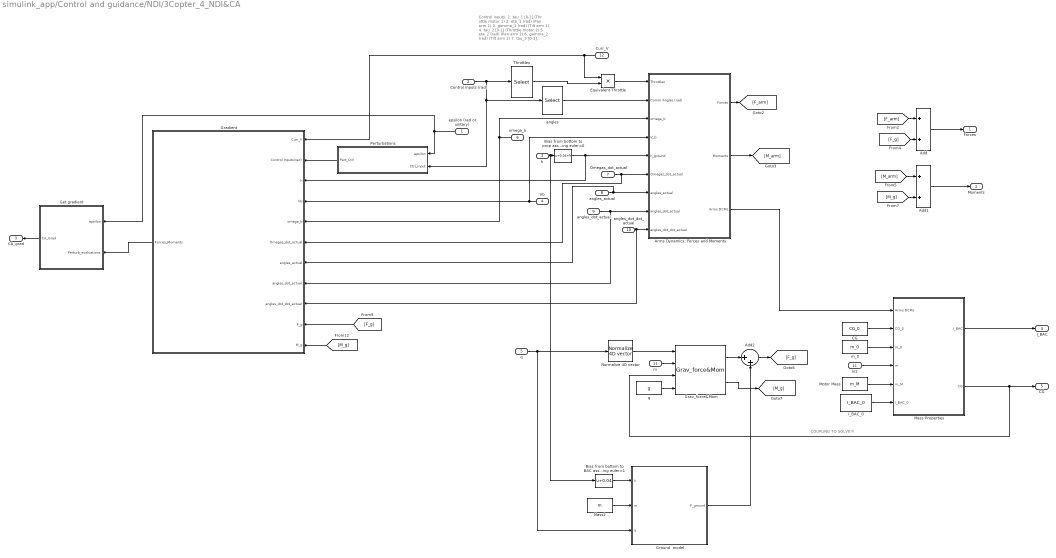
== system simulink_app/Control and guidance/NDI/3Copter_4_NDI&CA ==
  note: Control inputs:
      | 1. tau_1 [0-1] (Thr ottle motor 1)
      | 2. eta_1 (rad)  (Pan arm 1)
      | 3. gamma_1 (rad)  (Tilt arm 1)
      |
      | 4. tau_2 [0-1] (Throttle motor 2)
      | 5. eta_2 (rad)  (Pan arm 2)
      | 6. gamma_2 (rad)  (Tilt arm 2)
      |
      | 7. tau_3 [0-1] (Throttle motor 3)
      | 8. eta_3 (rad)  (Pan arm  3)
      | 9. gamma_3 (rad)  (Tilt arm 3)
  note: COUPLING TO SOLVE!!!
  "epsilon (rad or unitary) " : Inport
  Control Inputs (rad) : Inport  Port=2
  h : Inport  Port=3
  Vb : Inport  Port=4
  q : Inport  Port=5
  omega_b : Inport  Port=6
  Omegas_dot_actual : Inport  Port=7
  angles_actual : Inport  Port=8
  angles_dot_actual : Inport  Port=9
  angles_dot_dot_actual : Inport  Port=10
  " m" : Inport  Port=11
  Curr_V : Inport  Port=12
  Add : Sum
  Add1 : Sum
  Add2 : Sum  Inputs=|++
  Arms Dynamics: Forces and Moments : Subsystem  TreatAsAtomicUnit=on
  Bias from bottom to BAC assuming euler=1 : Bias  Bias=0.04
  Bias from bottom to prop assuming euler=0 : Bias  Bias=0.04+h
  CG : Constant  Value=CG_0
  Equivalent Throttle : Product  Inputs=**
  Get gradient : MATLAB Function  TreatAsAtomicUnit=on
  Gradient : Subsystem  TreatAsAtomicUnit=on
  Grav_force&Mom : XXCopter_Control/Grav_force&Mom
  Ground  model : Subsystem  TreatAsAtomicUnit=on
  I_BAC_0 : Constant  Value=I_BAC_0
  Mass Properties : Subsystem  TreatAsAtomicUnit=on
  Mass2 : Constant  Value=m
  Motor Mass : Constant  Value=m_M
  Normalize 4D vector : XXCopter/Normalize 4D vector
  Perturbations : MATLAB Function  TreatAsAtomicUnit=on
  Throttles : Selector  IndexMode=Zero-based  InputPortWidth=9  Indices=[0,3,6]
  "angles " : Selector  IndexMode=Zero-based  InputPortWidth=9  Indices=[1,2,4,5,7,8]
  "g " : Constant  Value=g
  m2 : InportShadow  Port=11
  m_0 : Constant  Value=m_0
  Forces : Outport
  Moments : Outport  Port=2
  CA_grad : Outport  Port=3
  I_BAC : Outport  Port=4
  "CG " : Outport  Port=5
  wires:
  Get gradient/1(CA_Grad) -> CA_grad/1
  "epsilon (rad or unitary) "/1 -> Perturbations/1(epsilon), Get gradient/1(epsilon)
  Perturbations/1(Pert_Ctrl) -> Gradient/2("Control Inputs(rad) ")
  Gradient/1(Forces_Moments) -> Get gradient/2(Perturb_evaluations)
  Mass Properties/1(I_BAC) -> I_BAC/1
  [F_g] -> Gradient/10(F_g)
  [M_g] -> Gradient/11(M_g)
  Normalize 4D vector/1 -> Grav_force&Mom/1
  angles_dot_actual/1 -> Arms Dynamics: Forces and Moments/8(angles_dot_actual), Gradient/8(angles_dot_actual)
  Omegas_dot_actual/1 -> Gradient/6(Omegas_dot_actual), Arms Dynamics: Forces and Moments/6(Omegas_dot_actual)
  Add1/1 -> Moments/1
  Curr_V/1 -> Gradient/1(Curr_V), Equivalent Throttle/1
  Equivalent Throttle/1 -> Arms Dynamics: Forces and Moments/1(Throttles)
  Mass Properties/2(CG) -> Grav_force&Mom/3, "CG "/1
  Add/1 -> Forces/1
  m2/1 -> Mass Properties/4(m)
  m_0/1 -> Mass Properties/3(m_0)
  I_BAC_0/1 -> Mass Properties/6(I_BAC_0)
  Motor Mass/1 -> Mass Properties/5(m_M)
  CG/1 -> Mass Properties/2(CG_0)
  Arms Dynamics: Forces and Moments/3(Arms DCMs) -> Mass Properties/1(Arms DCMs)
  Control Inputs (rad)/1 -> Throttles/1, Perturbations/2(Ctrl_input), "angles "/1
  Throttles/1 -> Equivalent Throttle/2
  [M_g] -> Add1/2
  [M_arm] -> Add1/1
  [F_g] -> Add/2
  [F_arm] -> Add/1
  Grav_force&Mom/2 -> [M_g]
  Arms Dynamics: Forces and Moments/2(Moments) -> [M_arm]
  Arms Dynamics: Forces and Moments/1(Forces) -> [F_arm]
  " m"/1 -> Grav_force&Mom/2
  omega_b/1 -> Gradient/5(omega_b), Arms Dynamics: Forces and Moments/3(omega_b)
  Vb/1 -> Arms Dynamics: Forces and Moments/4(V_b), Gradient/4(Vb)
  angles_actual/1 -> Gradient/7(angles_actual), Arms Dynamics: Forces and Moments/7(angles_actual)
  "angles "/1 -> Arms Dynamics: Forces and Moments/2(Comm Angles (rad))
  angles_dot_dot_actual/1 -> Gradient/9(angles_dot_dot_actual), Arms Dynamics: Forces and Moments/9(angles_dot_dot_actual)
  Bias from bottom to prop assuming euler=0/1 -> Arms Dynamics: Forces and Moments/5(h_ground), Gradient/3(h)
  Ground  model/1(F_ground) -> Add2/2
  q/1 -> Normalize 4D vector/1, Ground  model/3(q)
  Mass2/1 -> Ground  model/2(m)
  Bias from bottom to BAC assuming euler=1/1 -> Ground  model/1(h)
  h/1 -> Bias from bottom to prop assuming euler=0/1, Bias from bottom to BAC assuming euler=1/1
  Grav_force&Mom/1 -> Add2/1
  Add2/1 -> [F_g]
  "g "/1 -> Grav_force&Mom/4

== system simulink_app/Control and guidance/Otter Overactuated P Controller/Position Controller ==
  AWU : Inport
  X_e_x_ref : Inport  Port=2
  X_e_y_ref : Inport  Port=3
  X_e_z_ref : Inport  Port=4
  activation_bus : Inport  Port=5
  All_meas : Inport  Port=6
  init_cond : Inport  Port=7
  AWU1 : InportShadow
  AWU2 : InportShadow
  Bus Creator : BusCreator  Inputs=3
  Bus Creator1 : BusCreator  Inputs=3
  Bus Creator2 : BusCreator  Inputs=3
  Bus Selector : BusSelector  OutputSignals=Meas.Pos_meas_m
  Bus Selector1 : BusSelector  OutputSignals=pos_xy_init
  Bus Selector2 : BusSelector  OutputSignals=pos_xy_act
  Bus Selector3 : BusSelector  OutputSignals=alt_init
  Bus Selector4 : BusSelector  OutputSignals=alt_act
  Mux : Mux  Inputs=3
  Ref Model and PI Controller : XXCopter_Control/Ref Model and PI Controller  delta=0  tau=3  RisingSlewLimit=4  FallingSlewLimit=-4  K_f=0  K_a=1  Con_way=pro  omega_n=4  xi=0.5  Z1=-30  K_b=1.2  f_i=0.07  f_c=1
  Ref Model and PI Controller1 : XXCopter_Control/Ref Model and PI Controller  delta=0  tau=5  RisingSlewLimit=4  FallingSlewLimit=-4  K_f=0  K_a=1  Con_way=pro  omega_n=4  xi=0.5  Z1=-30  K_b=1  f_i=0.07  f_c=1
  Ref Model and PI Controller3 : XXCopter_Control/Ref Model and PI Controller  delta=0  tau=5  RisingSlewLimit=4  FallingSlewLimit=-4  K_f=0  K_a=1  Con_way=pro  omega_n=4  xi=0.5  Z1=-30  K_b=1  f_i=0.07  f_c=1
  Selector : Selector  InputPortWidth=3
  Selector1 : Selector  InputPortWidth=3  Indices=2
  Selector2 : Selector  InputPortWidth=3  Indices=3
  Selector3 : Selector  InputPortWidth=3
  Selector4 : Selector  InputPortWidth=3  Indices=2
  Selector5 : Selector  InputPortWidth=3  Indices=3
  Selector6 : Selector  InputPortWidth=2
  Selector7 : Selector  InputPortWidth=2  Indices=2
  Sum : Sum  Inputs=+-|
  Sum1 : Sum  Inputs=+-|
  Sum2 : Sum  Inputs=+-|
  Terminator1 : Terminator
  Terminator2 : Terminator
  Terminator3 : Terminator
  Ve des (m/s) : Outport
  wires:
  All_meas/1 -> Bus Selector/1
  Bus Selector/1 -> Selector/1, Selector1/1, Selector2/1  "<Pos_meas_m>"
  X_e_x_ref/1 -> Ref Model and PI Controller3/1
  Ref Model and PI Controller3/1 -> Mux/1
  Mux/1 -> Ve des (m/s)/1
  X_e_y_ref/1 -> Ref Model and PI Controller1/1
  X_e_z_ref/1 -> Ref Model and PI Controller/1
  Ref Model and PI Controller1/1 -> Mux/2
  Ref Model and PI Controller/1 -> Mux/3
  Ref Model and PI Controller3/2 -> Bus Creator/1  "X_ex_sf_dot"
  Ref Model and PI Controller3/3 -> Bus Creator/2, Sum/1  "X_ex_sf"
  Sum/1 -> Bus Creator/3  "X_ex_err"
  Bus Creator/1 -> Terminator2/1
  Bus Creator1/1 -> Terminator1/1
  Bus Creator2/1 -> Terminator3/1
  Ref Model and PI Controller3/4 -> Sum/2
  Ref Model and PI Controller1/2 -> Bus Creator1/1  "X_ey_sf_dot"
  Ref Model and PI Controller1/3 -> Sum1/1, Bus Creator1/2  "X_e_y_sf"
  Sum1/1 -> Bus Creator1/3  "X_ey_err"
  Ref Model and PI Controller1/4 -> Sum1/2
  Ref Model and PI Controller/2 -> Bus Creator2/1  "X_ez_sf_dot"
  Ref Model and PI Controller/3 -> Sum2/1, Bus Creator2/2  "X_ez_sf"
  Sum2/1 -> Bus Creator2/3  "X_ez_err"
  Ref Model and PI Controller/4 -> Sum2/2
  AWU/1 -> Selector3/1
  AWU1/1 -> Selector4/1
  AWU2/1 -> Selector5/1
  Selector3/1 -> Ref Model and PI Controller3/4
  Selector4/1 -> Ref Model and PI Controller1/4
  Selector5/1 -> Ref Model and PI Controller/4
  Selector2/1 -> Ref Model and PI Controller/2
  Selector1/1 -> Ref Model and PI Controller1/2
  Selector/1 -> Ref Model and PI Controller3/2
  init_cond/1 -> Bus Selector1/1, Bus Selector3/1
  activation_bus/1 -> Bus Selector4/1, Bus Selector2/1
  Bus Selector2/1 -> Ref Model and PI Controller1/Enable, Ref Model and PI Controller3/Enable  "<pos_xy_act>"
  Bus Selector1/1 -> Selector7/1, Selector6/1  "<pos_xy_init>"
  Selector6/1 -> Ref Model and PI Controller3/3
  Selector7/1 -> Ref Model and PI Controller1/3
  Bus Selector3/1 -> Ref Model and PI Controller/3  "<alt_init>"
  Bus Selector4/1 -> Ref Model and PI Controller/Enable  "<alt_act>"

== system simulink_app/Control and guidance/Otter Overactuated P Controller/Velocity Controller ==
  Vyaw_x_ref : Inport
  Vyaw_y_ref : Inport  Port=2
  Vyaw_z_ref : Inport  Port=3
  V_yaw_meas : Inport  Port=4
  activation_bus : Inport  Port=5
  Init_cond : Inport  Port=6
  Bus Creator : BusCreator
  Bus Creator1 : BusCreator
  Bus Creator2 : BusCreator
  Bus Selector1 : BusSelector  OutputSignals=vel_yaw_z_act
  Bus Selector2 : BusSelector  OutputSignals=vel_yaw_xy_act
  Bus Selector3 : BusSelector  OutputSignals=vel_yaw_xy_init
  Bus Selector4 : BusSelector  OutputSignals=vel_yaw_z_init
  Mux : Mux  Inputs=3
  Ref Model and P Controller p : XXCopter_Control/Ref Model and P Controller  tau=2  RisingSlewLimit=1  FallingSlewLimit=-1  K_f=0.5  K_b=1
  Ref Model and P Controller q : XXCopter_Control/Ref Model and P Controller  tau=2  RisingSlewLimit=1  FallingSlewLimit=-1  K_f=0.5  K_b=1
  Ref Model and P Controller r : XXCopter_Control/Ref Model and P Controller  tau=1  RisingSlewLimit=1  FallingSlewLimit=-1  K_f=0.4  K_b=8
  Selector : Selector  InputPortWidth=3
  Selector1 : Selector  InputPortWidth=3  Indices=2
  Selector2 : Selector  InputPortWidth=3  Indices=3
  Selector3 : Selector  InputPortWidth=2
  Selector4 : Selector  InputPortWidth=2  Indices=2
  Sum : Sum  Inputs=+-|
  Sum1 : Sum  Inputs=+-|
  Sum2 : Sum  Inputs=+-|
  Terminator1 : Terminator
  Terminator2 : Terminator
  Terminator3 : Terminator
  Acc_yaw des (m/s) : Outport
  wires:
  Ref Model and P Controller r/5 -> Bus Creator2/4  "K_b_Ve_z"
  Ref Model and P Controller r/4 -> Sum2/2
  Sum2/1 -> Bus Creator2/3  "Vez_err"
  Ref Model and P Controller r/3 -> Bus Creator2/2, Sum2/1  "Vez_sf"
  Ref Model and P Controller r/2 -> Bus Creator2/1  "Vez_sf_dot"
  Ref Model and P Controller q/5 -> Bus Creator1/4  "K_b_Vey"
  Ref Model and P Controller q/4 -> Sum1/2
  Sum1/1 -> Bus Creator1/3  "Vey_err"
  Ref Model and P Controller q/3 -> Bus Creator1/2, Sum1/1  "Ve_y_sf"
  Ref Model and P Controller q/2 -> Bus Creator1/1  "Vey_sf_dot"
  Ref Model and P Controller p/5 -> Bus Creator/4  "K_b_Vex"
  Ref Model and P Controller p/4 -> Sum/2
  Selector2/1 -> Ref Model and P Controller r/2
  Bus Creator2/1 -> Terminator3/1
  Bus Creator1/1 -> Terminator1/1
  Bus Creator/1 -> Terminator2/1
  Sum/1 -> Bus Creator/3  "Vex_err"
  Ref Model and P Controller p/3 -> Bus Creator/2, Sum/1  "Vex_sf"
  Ref Model and P Controller p/2 -> Bus Creator/1  "Vex_sf_dot"
  Ref Model and P Controller r/1 -> Mux/3
  Ref Model and P Controller q/1 -> Mux/2
  Vyaw_z_ref/1 -> Ref Model and P Controller r/1
  Selector1/1 -> Ref Model and P Controller q/2
  Vyaw_y_ref/1 -> Ref Model and P Controller q/1
  Mux/1 -> Acc_yaw des (m/s)/1
  Ref Model and P Controller p/1 -> Mux/1
  Vyaw_x_ref/1 -> Ref Model and P Controller p/1
  V_yaw_meas/1 -> Selector1/1, Selector/1, Selector2/1
  Selector/1 -> Ref Model and P Controller p/2
  activation_bus/1 -> Bus Selector1/1, Bus Selector2/1
  Bus Selector2/1 -> Ref Model and P Controller q/Enable, Ref Model and P Controller p/Enable  "<vel_yaw_xy_act>"
  Bus Selector1/1 -> Ref Model and P Controller r/Enable  "<vel_yaw_z_act>"
  Init_cond/1 -> Bus Selector4/1, Bus Selector3/1
  Bus Selector3/1 -> Selector3/1, Selector4/1  "<vel_yaw_xy_init>"
  Selector3/1 -> Ref Model and P Controller p/3
  Selector4/1 -> Ref Model and P Controller q/3
  Bus Selector4/1 -> Ref Model and P Controller r/3  "<vel_yaw_z_init>"

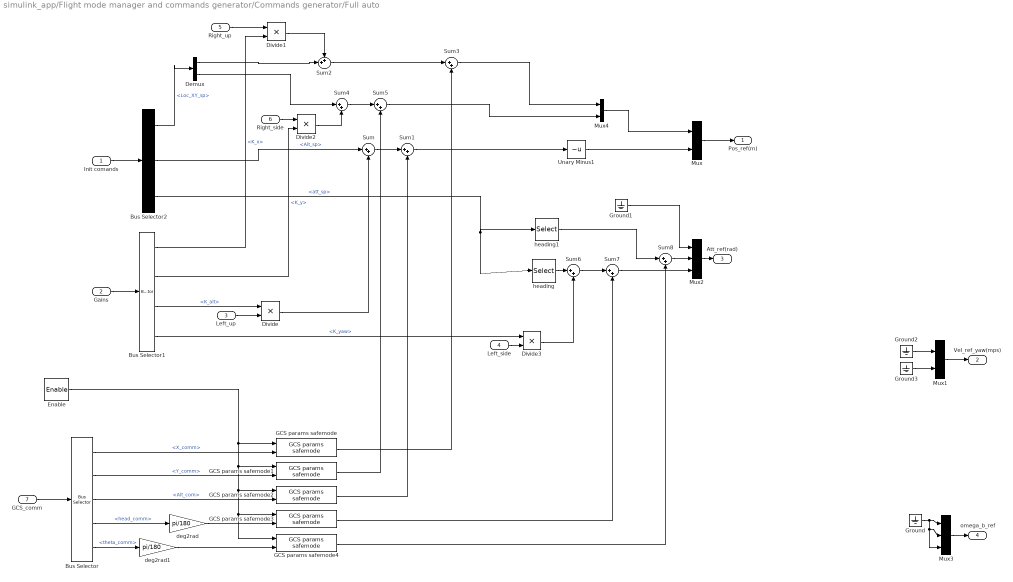
== system simulink_app/Flight mode manager and commands generator/Commands generator/Full auto ==
  Init comands : Inport
  Gains : Inport  Port=2
  Left_up : Inport  Port=3
  Left_side : Inport  Port=4
  Right_up : Inport  Port=5
  Right_side : Inport  Port=6
  GCS_comm : Inport  Port=7
  Enable : EnablePort  StatesWhenEnabling=reset  ShowOutputPort=on
  Bus Selector : BusSelector  OutputSignals=X_comm,Y_comm,Alt_com,head_comm,theta_comm
  Bus Selector1 : BusSelector  OutputSignals=K_x,K_y,K_alt,K_yaw
  Bus Selector2 : BusSelector  OutputSignals=Loc_XY_sp,Alt_sp,att_sp
  Demux : Demux  Outputs=2
  Divide{,1..3} (4 alike) : Product  Inputs=**
  GCS params safemode{,1..4} (5 alike) : XXCopter_Control/GCS params safemode
  Ground{,1..3} (4 alike) : Ground
  Mux : Mux  Inputs=[2,1]
  Mux1 : Mux  Inputs=[2,1]
  Mux2 : Mux  Inputs=3
  Mux3 : Mux  Inputs=3
  Mux4 : Mux  Inputs=2
  Sum{,1,3..8} (8 alike) : Sum  Inputs=|++
  Sum2 : Sum  Inputs=++|
  Unary Minus1 : UnaryMinus
  deg2rad : Gain  Gain=pi/180
  deg2rad1 : Gain  Gain=pi/180
  heading : Selector  InputPortWidth=3  Indices=3
  heading1 : Selector  InputPortWidth=3  Indices=2
  Pos_ref(m) : Outport
  Vel_ref_yaw(mps) : Outport  Port=2
  Att_ref(rad) : Outport  Port=3
  omega_b_ref : Outport  Port=4
  wires:
  Bus Selector2/2 -> Sum/1  "<Alt_sp>"
  Divide/1 -> Sum/2
  Sum/1 -> Sum1/1
  GCS params safemode2/1 -> Sum1/2
  Sum1/1 -> Unary Minus1/1
  GCS_comm/1 -> Bus Selector/1
  Bus Selector/1 -> GCS params safemode/2  "<X_comm>"
  Bus Selector/2 -> GCS params safemode1/2  "<Y_comm>"
  Bus Selector/3 -> GCS params safemode2/2  "<Alt_com>"
  Bus Selector/4 -> deg2rad/1  "<head_comm>"
  Mux1/1 -> Vel_ref_yaw(mps)/1
  Mux/1 -> Pos_ref(m)/1
  Mux2/1 -> Att_ref(rad)/1
  Unary Minus1/1 -> Mux/2
  Ground/1 -> Mux3/3, Mux3/2, Mux3/1
  Ground1/1 -> Mux2/1
  Ground2/1 -> Mux1/1
  Ground3/1 -> Mux1/2
  Mux4/1 -> Mux/1
  Mux3/1 -> omega_b_ref/1
  Gains/1 -> Bus Selector1/1
  Init comands/1 -> Bus Selector2/1
  Bus Selector1/3 -> Divide/1  "<K_alt>"
  Left_up/1 -> Divide/2
  Bus Selector2/1 -> Demux/1  "<Loc_XY_sp>"
  Sum2/1 -> Sum3/1
  Sum3/1 -> Mux4/1
  GCS params safemode/1 -> Sum3/2
  Demux/1 -> Sum2/2
  Right_up/1 -> Divide1/1
  Bus Selector1/1 -> Divide1/2  "<K_x>"
  Divide1/1 -> Sum2/1
  Sum4/1 -> Sum5/1
  GCS params safemode1/1 -> Sum5/2
  Sum5/1 -> Mux4/2
  Divide2/1 -> Sum4/2
  Demux/2 -> Sum4/1
  Right_side/1 -> Divide2/1
  Bus Selector1/2 -> Divide2/2  "<K_y>"
  Sum6/1 -> Sum7/1
  Sum7/1 -> Mux2/3
  GCS params safemode3/1 -> Sum7/2
  heading/1 -> Sum6/1
  Bus Selector2/3 -> heading1/1, heading/1  "<att_sp>"
  Bus Selector1/4 -> Divide3/1  "<K_yaw>"
  Left_side/1 -> Divide3/2
  Divide3/1 -> Sum6/2
  Bus Selector/5 -> deg2rad1/1  "<theta_comm>"
  GCS params safemode4/1 -> Sum8/2
  heading1/1 -> Sum8/1
  Sum8/1 -> Mux2/2
  deg2rad/1 -> GCS params safemode3/2
  deg2rad1/1 -> GCS params safemode4/2
  Enable/1 -> GCS params safemode4/1, GCS params safemode3/1, GCS params safemode2/1, GCS params safemode1/1, GCS params safemode/1

== system simulink_app/Flight mode manager and commands generator/Commands generator/Home ==
  Init comands : Inport
  Gains : Inport  Port=2
  Left_up : Inport  Port=3
  Left_side : Inport  Port=4
  Right_up : Inport  Port=5
  Right_side : Inport  Port=6
  GCS_comm : Inport  Port=7
  Enable : EnablePort  StatesWhenEnabling=reset
  Bus Selector2 : BusSelector  OutputSignals=Loc_XY_sp,Alt_sp,att_sp
  Ground{,1..3} (4 alike) : Ground
  Mux : Mux  Inputs=[2,1]
  Mux1 : Mux  Inputs=[2,1]
  Mux2 : Mux  Inputs=3
  Selector : Selector  InputPortWidth=3  Indices=3
  Terminator{,1..5} (6 alike) : Terminator
  Unary Minus : UnaryMinus
  Pos_ref(m) : Outport
  Vel_ref_yaw(mps) : Outport  Port=2
  Att_ref(rad) : Outport  Port=3
  omega_b_ref : Outport  Port=4
  wires:
  Mux1/1 -> Vel_ref_yaw(mps)/1
  Mux2/1 -> Att_ref(rad)/1
  Ground1/1 -> Mux2/2, Mux2/1
  Ground2/1 -> Mux1/1
  Ground3/1 -> Mux1/2
  Mux/1 -> Pos_ref(m)/1
  Ground/1 -> omega_b_ref/1
  Gains/1 -> Terminator/1
  Right_up/1 -> Terminator1/1
  Left_up/1 -> Terminator2/1
  Left_side/1 -> Terminator3/1
  Right_side/1 -> Terminator4/1
  GCS_comm/1 -> Terminator5/1
  Init comands/1 -> Bus Selector2/1
  Bus Selector2/1 -> Mux/1  "<Loc_XY_sp>"
  Bus Selector2/2 -> Unary Minus/1  "<Alt_sp>"
  Unary Minus/1 -> Mux/2
  Selector/1 -> Mux2/3
  Bus Selector2/3 -> Selector/1  "<att_sp>"

== system simulink_app/Flight mode manager and commands generator/Commands generator/Land  ==
  Init comands : Inport
  Gains : Inport  Port=2
  Left_up : Inport  Port=3
  Left_side : Inport  Port=4
  Right_up : Inport  Port=5
  Right_side : Inport  Port=6
  GCS_comm : Inport  Port=7
  Enable : EnablePort  StatesWhenEnabling=reset
  Bus Selector2 : BusSelector  OutputSignals=Loc_XY_sp,Alt_sp,att_sp
  Ground{,1..3} (4 alike) : Ground
  Mux : Mux  Inputs=[2,1]
  Mux1 : Mux  Inputs=[2,1]
  Mux2 : Mux  Inputs=3
  Selector : Selector  InputPortWidth=3  Indices=3
  Terminator{,1..5} (6 alike) : Terminator
  Unary Minus : UnaryMinus
  Pos_ref(m) : Outport
  Vel_ref_yaw(mps) : Outport  Port=2
  Att_ref(rad) : Outport  Port=3
  omega_b_ref : Outport  Port=4
  wires:
  Mux1/1 -> Vel_ref_yaw(mps)/1
  Mux2/1 -> Att_ref(rad)/1
  Ground/1 -> omega_b_ref/1
  Ground1/1 -> Mux2/2, Mux2/1
  Ground2/1 -> Mux1/1
  Ground3/1 -> Mux1/2
  Mux/1 -> Pos_ref(m)/1
  Gains/1 -> Terminator/1
  Right_up/1 -> Terminator1/1
  Left_up/1 -> Terminator2/1
  Left_side/1 -> Terminator3/1
  Right_side/1 -> Terminator4/1
  GCS_comm/1 -> Terminator5/1
  Init comands/1 -> Bus Selector2/1
  Bus Selector2/1 -> Mux/1  "<Loc_XY_sp>"
  Bus Selector2/2 -> Unary Minus/1  "<Alt_sp>"
  Unary Minus/1 -> Mux/2
  Selector/1 -> Mux2/3
  Bus Selector2/3 -> Selector/1  "<att_sp>"

== system simulink_app/Flight mode manager and commands generator/Commands generator/Man_ctrl ==
  Init comands : Inport
  Gains : Inport  Port=2
  Left_up : Inport  Port=3
  Left_side : Inport  Port=4
  Right_up : Inport  Port=5
  Right_side : Inport  Port=6
  GCS_comm : Inport  Port=7
  Enable : EnablePort  StatesWhenEnabling=reset
  Bus Selector1 : BusSelector  OutputSignals=K_vz,K_p,K_q,K_r
  Divide{1..4} (4 alike) : Product  Inputs=**
  Ground{1..2,4..5} (4 alike) : Ground
  Mux : Mux  Inputs=[2,1]
  Mux1 : Mux  Inputs=[2,1]
  Mux2 : Mux  Inputs=3
  Mux3 : Mux  Inputs=3
  Terminator : Terminator
  Terminator1 : Terminator
  Unary Minus : UnaryMinus
  Unary Minus1 : UnaryMinus
  Pos_ref(m) : Outport
  Vel_ref_yaw(mps) : Outport  Port=2
  Att_ref(rad) : Outport  Port=3
  omega_b_ref : Outport  Port=4
  wires:
  Mux1/1 -> Vel_ref_yaw(mps)/1
  Mux2/1 -> Att_ref(rad)/1
  Ground5/1 -> Mux/2
  Ground1/1 -> Mux2/3, Mux2/2, Mux2/1
  Ground2/1 -> Mux1/1
  Unary Minus1/1 -> Mux1/2
  Mux/1 -> Pos_ref(m)/1
  Mux3/1 -> omega_b_ref/1
  GCS_comm/1 -> Terminator/1
  Init comands/1 -> Terminator1/1
  Gains/1 -> Bus Selector1/1
  Bus Selector1/1 -> Divide1/2  "<K_vz>"
  Left_up/1 -> Divide1/1
  Ground4/1 -> Mux/1
  Bus Selector1/2 -> Divide2/1  "<K_p>"
  Right_side/1 -> Divide2/2
  Bus Selector1/3 -> Divide3/1  "<K_q>"
  Right_up/1 -> Divide3/2
  Bus Selector1/4 -> Divide4/1  "<K_r>"
  Left_side/1 -> Divide4/2
  Divide3/1 -> Unary Minus/1
  Divide2/1 -> Mux3/1
  Unary Minus/1 -> Mux3/2
  Divide4/1 -> Mux3/3
  Divide1/1 -> Unary Minus1/1

== system simulink_app/Flight mode manager and commands generator/Commands generator/Off//Ready ==
  Init comands : Inport
  Gains : Inport  Port=2
  Left_up : Inport  Port=3
  Left_side : Inport  Port=4
  Right_up : Inport  Port=5
  Right_side : Inport  Port=6
  GCS_comm : Inport  Port=7
  Enable : EnablePort  StatesWhenEnabling=reset
  Ground{,1..3} (4 alike) : Ground
  Terminator{,1..6} (7 alike) : Terminator
  Pos_ref(m) : Outport
  Vel_ref_yaw(mps) : Outport  Port=2
  Att_ref(rad) : Outport  Port=3
  omega_b_ref : Outport  Port=4
  wires:
  Gains/1 -> Terminator/1
  Right_up/1 -> Terminator1/1
  Left_up/1 -> Terminator2/1
  Left_side/1 -> Terminator3/1
  Right_side/1 -> Terminator4/1
  GCS_comm/1 -> Terminator5/1
  Ground/1 -> Pos_ref(m)/1
  Ground1/1 -> Att_ref(rad)/1
  Ground2/1 -> Vel_ref_yaw(mps)/1
  Ground3/1 -> omega_b_ref/1
  Init comands/1 -> Terminator6/1

== system simulink_app/Flight mode manager and commands generator/Commands generator/Stab ==
  Init comands : Inport
  Gains : Inport  Port=2
  Left_up : Inport  Port=3
  Left_side : Inport  Port=4
  Right_up : Inport  Port=5
  Right_side : Inport  Port=6
  GCS_comm : Inport  Port=7
  Enable : EnablePort  StatesWhenEnabling=reset  ShowOutputPort=on
  Bus Selector : BusSelector  OutputSignals=Vz_yaw_comm,head_comm
  Bus Selector1 : BusSelector  OutputSignals=K_vz,K_phi,K_theta,K_yaw
  Bus Selector2 : BusSelector  OutputSignals=Vel_yaw_z_sp,att_sp
  Divide{1..4} (4 alike) : Product  Inputs=**
  GCS params safemode2 : XXCopter_Control/GCS params safemode
  GCS params safemode3 : XXCopter_Control/GCS params safemode
  Ground{,2..4} (4 alike) : Ground
  Mux : Mux  Inputs=[2,1]
  Mux1 : Mux  Inputs=[2,1]
  Mux2 : Mux  Inputs=3
  Selector : Selector  InputPortWidth=3  Indices=3
  Sum{3,6,8..9} (4 alike) : Sum  Inputs=|++
  Unary Minus : UnaryMinus
  Unary Minus1 : UnaryMinus
  deg2rad1 : Gain  Gain=pi/180
  Pos_ref(m) : Outport
  Vel_ref_yaw(mps) : Outport  Port=2
  Att_ref(rad) : Outport  Port=3
  omega_b_ref : Outport  Port=4
  wires:
  Mux1/1 -> Vel_ref_yaw(mps)/1
  Mux2/1 -> Att_ref(rad)/1
  Mux/1 -> Pos_ref(m)/1
  Ground/1 -> omega_b_ref/1
  GCS_comm/1 -> Bus Selector/1
  Bus Selector/1 -> GCS params safemode2/2  "<Vz_yaw_comm>"
  Bus Selector/2 -> deg2rad1/1  "<head_comm>"
  deg2rad1/1 -> GCS params safemode3/2
  Bus Selector2/1 -> Sum3/1  "<Vel_yaw_z_sp>"
  Gains/1 -> Bus Selector1/1
  Init comands/1 -> Bus Selector2/1
  Sum3/1 -> Sum6/1
  Divide3/1 -> Sum3/2
  Left_up/1 -> Divide3/2
  Ground4/1 -> Mux/1
  GCS params safemode2/1 -> Sum6/2
  Sum6/1 -> Unary Minus/1
  Right_up/1 -> Divide1/1
  Right_side/1 -> Divide2/1
  Sum8/1 -> Sum9/1
  Selector/1 -> Sum8/1
  Bus Selector2/2 -> Selector/1  "<att_sp>"
  Left_side/1 -> Divide4/2
  Divide4/1 -> Sum8/2
  Sum9/1 -> Mux2/3
  GCS params safemode3/1 -> Sum9/2
  Ground2/1 -> Mux1/1
  Unary Minus/1 -> Mux1/2
  Bus Selector1/1 -> Divide3/1  "<K_vz>"
  Bus Selector1/4 -> Divide4/1  "<K_yaw>"
  Bus Selector1/2 -> Divide2/2  "<K_phi>"
  Bus Selector1/3 -> Divide1/2  "<K_theta>"
  Enable/1 -> GCS params safemode3/1, GCS params safemode2/1
  Ground3/1 -> Mux/2
  Divide2/1 -> Mux2/1
  Divide1/1 -> Unary Minus1/1
  Unary Minus1/1 -> Mux2/2
